simulink model "RL_TTS3_Controller_Blank"  (R2019b)
settings: Solver=FixedStepAuto  StartTime=0.0  StopTime=1900  FixedStep=0.01  RelTol=1e-3
PostLoadFcn:
  | if any(exist('dsrtsu_mdlpostloadfcn', 'file') ~= 0), dsrtsu_mdlpostloadfcn('Execute', bdroot); end
libraries: simulink x1
settings Model: DSRTSU_INTERNAL_RTI_VER=550  DSRTSU_INTERNAL_RTI_TYPE=rti1104  RTICANMMDATA=struct('GeneralSetupData',struct('modelroot','E:\Will\RemoteLabs\TTS3\HostPC','generalsettings',struct('filesettings',struct('destfolder',struct('Name','RTICANMM_FILES','Check',1),'buildfolder',struct('Name','.','Check',1),'AbsDestfolder',struct('Name','E:\Will\RemoteLabs\TTS3\HostPC\RTICANMM_FILES'),'AbsBuildfolder',struct('Name','E:\Will\RemoteLabs\TTS3\HostPC'))),'options',struct('addpaths',1,'rmpaths',1,'addtrcexclusion',true,'cannavigator',struct('checkmonitoring',0),'show_usrtrc',0,'use_usrtrc',0),'advanced',struct('options',ones(1,100)),'MPSetup',{{}},'RTI',struct('Type','RTI1104','Ver','7.13','Date','02-Nov-2019'),'modelname','TTS3_Controller_Test_OL','block','TTS3_Controller_Test_OL'))  DSRTSU_INTERNAL_RTIFPGA=150  Creator=whendrix  LastModifiedBy=Bart
settings OptimizationCC: BlockReduction=off  OptimizeBlockIOStorage=off  BufferReuse=off  GlobalBufferReuse=off  ExpressionFolding=off  LocalBlockOutputs=off  OptimizeDataStoreBuffers=off  BusAssignmentInplaceUpdate=off
settings DebuggingCC: BusObjectLabelMismatch=none
settings HardwareCC: ProdBitPerPointer=32  ProdBitPerSizeT=32  ProdBitPerPtrDiffT=32  ProdLargestAtomicInteger=Integer  ProdEndianess=BigEndian  ProdWordSize=32  ProdHWDeviceType=Custom Processor->Custom  TargetIntDivRoundTo=Zero  TargetEndianess=BigEndian  TargetHWDeviceType=Custom Processor->Custom
settings ModelReferenceCC: ModelReferenceNumInstancesAllowed=Single  ModelReferenceMinAlgLoopOccurrences=on
settings SFSimCC: MATLABDynamicMemAlloc=off  CustomCodeUndefinedFunction=UseInterfaceOnly
settings RTWCC: Description=dSPACE DS1104 Hardware Platform  SystemTargetFile=rti1104.tlc  MakeCommand=make_rti  TemplateMakefile=rti1104.tmf
settings CodeAppCC: MaxIdLength=63
settings STFCustomTargetCC: ParMdlRefBuildCompliant=on  SystemTargetFile=rti1104.tlc
settings GRTTargetCC: TargetLangStandard=C89/C90 (ANSI)  CompOptLevelCompliant=off  ConcurrentExecutionCompliant=off  CombineOutputUpdateFcns=off  MatFileLogging=off  CPPClassGenCompliant=off  UseToolchainInfoCompliant=off

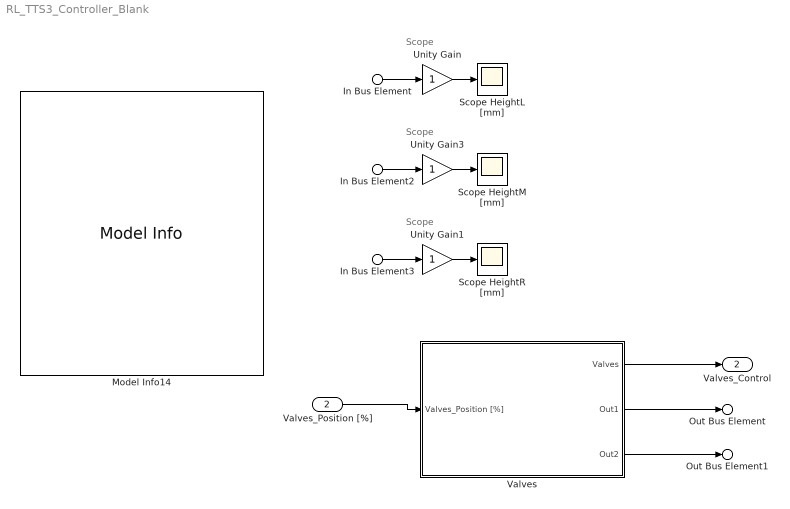
== system RL_TTS3_Controller_Blank ==
  note: Scope
  note: Scope
  note: Scope
  In Bus Element : Inport  PortName=Heights [mm]  Element=Left
  In Bus Element2 : Inport  PortName=Heights [mm]  Element=Middle
  In Bus Element3 : Inport  PortName=Heights [mm]  Element=Right
  Valves_Position [%] : Inport  Port=2  OutDataTypeStr=Bus: ValvesSOCI
  Model Info14 : simulink/Model-Wide Utilities/Model Info  Frame=on  DisplayStringWithTags=|  HorizontalTextAlignment=Left  LeftAlignmentValue=0.02
      | Start model for the "Three Tank"
      | experiment on the "Three Tank" setup.
      | Version: 1.0
      | 
      | 
      | INFORMATION
      | ----------------------
      | 
      | Unity Gain block before Scope is needed for
      | RemoteLabs compatebility. 
      | Do not modify or remove!
      | 
      | Pump range:
      | 0 to 0.102 [l/s]
      | 
      | The 5 Valves are labeled according 
      | to their position:
      | 
      |    LM  MR
      |      X     X
      |  X      X      X
      | LD    MD   RD
      | 
      | L = Left
      | M = Middle
      | R = Right
      | D = Down
  Scope HeightL [mm] : Scope
  Scope HeightM [mm] : Scope
  Scope HeightR [mm] : Scope
  Unity Gain : Gain
  Unity Gain1 : Gain
  Unity Gain3 : Gain
  Valves : Subsystem  TreatAsAtomicUnit=on
  Out Bus Element : Outport  VectorParamsAs1DForOutWhenUnconnected=off  PortName=Pumps [l/s]  Element=Left
  Out Bus Element1 : Outport  VectorParamsAs1DForOutWhenUnconnected=off  PortName=Pumps [l/s]  Element=Right
  Valves_Control : Outport  Port=2  OutDataTypeStr=Bus: ValvesSICO  VectorParamsAs1DForOutWhenUnconnected=off
  wires:
  Unity Gain3/1 -> Scope HeightM [mm]/1
  Unity Gain1/1 -> Scope HeightR [mm]/1
  In Bus Element/1 -> Unity Gain/1
  In Bus Element2/1 -> Unity Gain3/1
  In Bus Element3/1 -> Unity Gain1/1
  Valves/1(Valves) -> Valves_Control/1
  Valves_Position [%]/1 -> Valves/1(Valves_Position [%])
  Unity Gain/1 -> Scope HeightL [mm]/1
  Valves/2(Out1) -> Out Bus Element/1
  Valves/3(Out2) -> Out Bus Element1/1

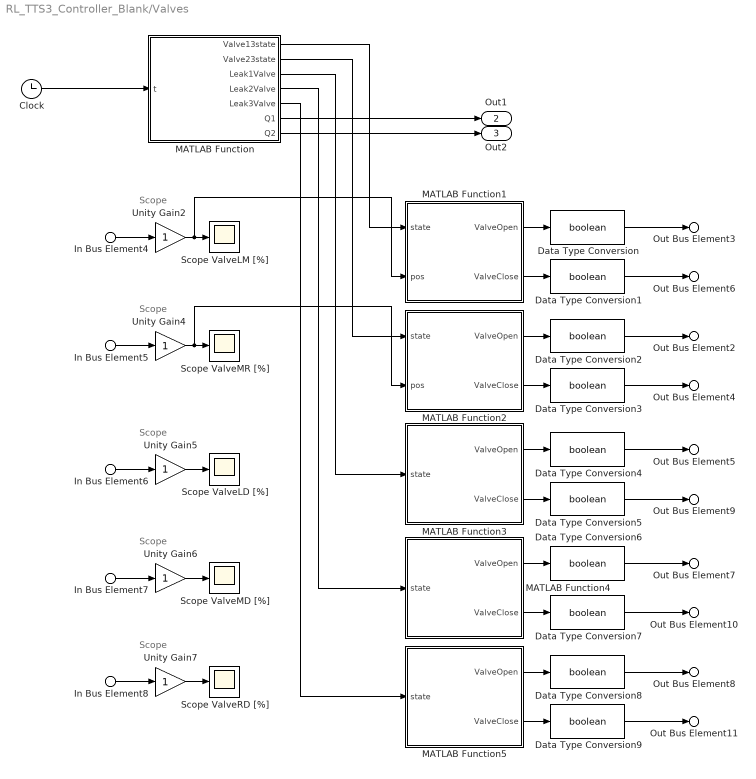
== system RL_TTS3_Controller_Blank/Valves ==
  note: Scope
  note: Scope
  note: Scope
  note: Scope
  note: Scope
  In Bus Element4 : Inport  PortName=Valves_Position [%]  Element=LeftMiddle
  In Bus Element5 : Inport  PortName=Valves_Position [%]  Element=MiddleRight
  In Bus Element6 : Inport  PortName=Valves_Position [%]  Element=LeftDown
  In Bus Element7 : Inport  PortName=Valves_Position [%]  Element=MiddleDown
  In Bus Element8 : Inport  PortName=Valves_Position [%]  Element=RightDown
  Clock : Clock
      settings: Decimation=100
  Data Type Conversion{,1..9} (10 alike) : DataTypeConversion  OutDataTypeStr=boolean
  MATLAB Function : MATLAB Function  TreatAsAtomicUnit=on
  MATLAB Function1 : MATLAB Function  TreatAsAtomicUnit=on
  MATLAB Function2 : MATLAB Function  TreatAsAtomicUnit=on
  MATLAB Function3 : MATLAB Function  TreatAsAtomicUnit=on
  MATLAB Function4 : MATLAB Function  TreatAsAtomicUnit=on
  MATLAB Function5 : MATLAB Function  TreatAsAtomicUnit=on
  Scope ValveLD [%] : Scope
  Scope ValveLM [%] : Scope
  Scope ValveMD [%] : Scope
  Scope ValveMR [%] : Scope
  Scope ValveRD [%] : Scope
  Unity Gain{2,4..7} (5 alike) : Gain
  Out Bus Element8 : Outport  VectorParamsAs1DForOutWhenUnconnected=off  PortName=Valves  Element=RightDown.Open
  Out Bus Element11 : Outport  VectorParamsAs1DForOutWhenUnconnected=off  PortName=Valves  Element=RightDown.Close
  Out Bus Element5 : Outport  VectorParamsAs1DForOutWhenUnconnected=off  PortName=Valves  Element=LeftDown.Open
  Out Bus Element9 : Outport  VectorParamsAs1DForOutWhenUnconnected=off  PortName=Valves  Element=LeftDown.Close
  Out Bus Element7 : Outport  VectorParamsAs1DForOutWhenUnconnected=off  PortName=Valves  Element=MiddleDown.Open
  Out Bus Element10 : Outport  VectorParamsAs1DForOutWhenUnconnected=off  PortName=Valves  Element=MiddleDown.Close
  Out Bus Element2 : Outport  VectorParamsAs1DForOutWhenUnconnected=off  PortName=Valves  Element=MiddleRight.Open
  Out Bus Element4 : Outport  VectorParamsAs1DForOutWhenUnconnected=off  PortName=Valves  Element=MiddleRight.Close
  Out Bus Element3 : Outport  VectorParamsAs1DForOutWhenUnconnected=off  PortName=Valves  Element=LeftMiddle.Open
  Out Bus Element6 : Outport  VectorParamsAs1DForOutWhenUnconnected=off  PortName=Valves  Element=LeftMiddle.Close
  Out1 : Outport  Port=2
  Out2 : Outport  Port=3
  wires:
  In Bus Element5/1 -> Unity Gain4/1
  In Bus Element4/1 -> Unity Gain2/1
  In Bus Element7/1 -> Unity Gain6/1
  Unity Gain6/1 -> Scope ValveMD [%]/1
  In Bus Element6/1 -> Unity Gain5/1
  In Bus Element8/1 -> Unity Gain7/1
  Unity Gain7/1 -> Scope ValveRD [%]/1
  Unity Gain4/1 -> MATLAB Function2/2(pos), Scope ValveMR [%]/1
  Unity Gain5/1 -> Scope ValveLD [%]/1
  Unity Gain2/1 -> MATLAB Function1/2(pos), Scope ValveLM [%]/1
  Data Type Conversion/1 -> Out Bus Element3/1
  Data Type Conversion1/1 -> Out Bus Element6/1
  Data Type Conversion2/1 -> Out Bus Element2/1
  Data Type Conversion3/1 -> Out Bus Element4/1
  Data Type Conversion4/1 -> Out Bus Element5/1
  Data Type Conversion5/1 -> Out Bus Element9/1
  Data Type Conversion6/1 -> Out Bus Element7/1
  Data Type Conversion7/1 -> Out Bus Element10/1
  Data Type Conversion8/1 -> Out Bus Element8/1
  Data Type Conversion9/1 -> Out Bus Element11/1
  Clock/1 -> MATLAB Function/1(t)
  MATLAB Function1/1(ValveOpen) -> Data Type Conversion/1
  MATLAB Function1/2(ValveClose) -> Data Type Conversion1/1
  MATLAB Function/1(Valve13state) -> MATLAB Function1/1(state)
  MATLAB Function2/1(ValveOpen) -> Data Type Conversion2/1
  MATLAB Function2/2(ValveClose) -> Data Type Conversion3/1
  MATLAB Function/2(Valve23state) -> MATLAB Function2/1(state)
  MATLAB Function3/1(ValveOpen) -> Data Type Conversion4/1
  MATLAB Function3/2(ValveClose) -> Data Type Conversion5/1
  MATLAB Function/3(Leak1Valve) -> MATLAB Function3/1(state)
  MATLAB Function4/1(ValveOpen) -> Data Type Conversion6/1
  MATLAB Function4/2(ValveClose) -> Data Type Conversion7/1
  MATLAB Function5/1(ValveOpen) -> Data Type Conversion8/1
  MATLAB Function5/2(ValveClose) -> Data Type Conversion9/1
  MATLAB Function/5(Leak3Valve) -> MATLAB Function5/1(state)
  MATLAB Function/4(Leak2Valve) -> MATLAB Function4/1(state)
  MATLAB Function/6(Q1) -> Out1/1
  MATLAB Function/7(Q2) -> Out2/1

== matlab function RL_TTS3_Controller_Blank/Valves/MATLAB Function1 ==
  data: state input; ValveOpen output; ValveClose output; pos input
function [ValveOpen, ValveClose] = Valve13(state,pos)
statepos = state(2);
state = state(1);

switch state
    case 0
        ValveOpen = false;
        ValveClose = true;
    case 1
        if(pos<statepos)
            ValveOpen = true;
            ValveClose = false;
        elseif(pos>=statepos)
            % semiopen poistion
            ValveOpen = false;
            ValveClose = false;
        end
    case 2
        ValveOpen = false;
        ValveClose = false;
    case 3
        ValveOpen = true;
        ValveClose = false;
    otherwise
        0;
end
end

== matlab function RL_TTS3_Controller_Blank/Valves/MATLAB Function ==
  data: t input; Valve13state output; Valve23state output; Leak1Valve output; Leak2Valve output; Leak3Valve output; Q1 output; Q2 output
function [Valve13state,Valve23state, Leak1Valve, Leak2Valve, Leak3Valve, Q1,Q2] = FSM(t)

percentageOpen = 20;
tankToTest = 2;

% state nr:
% 0: all valves closed
% 1: let valves go from a initial position to a percentage
% 2: do nothing
% 3: all valves 100% open

if(tankToTest==1)
    if(t<=90)
        % state 0
        Valve13state = [0 0];
        Valve23state = [0 0];
        Leak1Valve = 0;
        Leak2Valve = 0;
        Leak3Valve = 0;
        Q1 = 0.1;
        Q2 = 0;
        
    elseif (t>90 && t<=100)
        % state 1
        Valve13state = [1 percentageOpen];
        Valve23state = [1 0];
        Leak1Valve = 1;
        Leak2Valve = 1;
        Leak3Valve = 1;
        Q1 = 0;
        Q2 = 0;
        
    elseif (t>100)
        % state 2: observe
        Valve13state = [2 0];
        Valve23state = [2 0];
        Leak1Valve = 2;
        Leak2Valve = 2;
        Leak3Valve = 2;
        Q1 = 0;
        Q2 = 0;
    end
    
    
end

if(tankToTest==2)
    if(t<=80)
        % state 0
        Valve13state = [0 0];
        Valve23state = [0 0];
        Leak1Valve = 0;
        Leak2Valve = 0;
        Leak3Valve = 0;
        Q1 = 0;
        Q2 = 0.1;
        
    elseif (t>80 && t<=90)
        % state 1
        Valve13state = [1 0];
        Valve23state = [1 percentageOpen];
        Leak1Valve = 1;
        Leak2Valve = 1;
        Leak3Valve = 1;
        Q1 = 0;
        Q2 = 0;
        
    elseif (t>90)
        % state 2: observe
        Valve13state = [2 0];
        Valve23state = [2 0];
        Leak1Valve = 2;
        Leak2Valve = 2;
        Leak3Valve = 2;
        Q1 = 0;
        Q2 = 0;
    end
    
    
end
end

== matlab function RL_TTS3_Controller_Blank/Valves/MATLAB Function2 ==
  data: state input; ValveOpen output; ValveClose output; pos input
function [ValveOpen, ValveClose] = Valve32(state,pos)
statepos = state(2);
state = state(1);

switch state
    case 0
        ValveOpen = false;
        ValveClose = true;
    case 1
        if(pos<statepos)
            ValveOpen = true;
            ValveClose = false;
        elseif(pos>=statepos)
            % semiopen poistion
            ValveOpen = false;
            ValveClose = false;
        end
    case 2
        ValveOpen = false;
        ValveClose = false;
    case 3
        ValveOpen = true;
        ValveClose = false;
    otherwise
        0;
end
end

== matlab function RL_TTS3_Controller_Blank/Valves/MATLAB Function3 ==
  data: state input; ValveOpen output; ValveClose output
function [ValveOpen, ValveClose] = Leak1Valve(state)
switch state
    case 0
        ValveOpen = false;
        ValveClose = true;
    case 1
        ValveOpen = false;
        ValveClose = true;
    case 2
        ValveOpen = false;
        ValveClose = true;
    case 3
        ValveOpen = true;
        ValveClose = false;
    otherwise
        0;
end
end

== matlab function RL_TTS3_Controller_Blank/Valves/MATLAB Function4 ==
  data: state input; ValveOpen output; ValveClose output
function [ValveOpen, ValveClose] = Leak2Valve(state)
switch state
    case 0
        ValveOpen = false;
        ValveClose = true;
    case 1
        ValveOpen = false;
        ValveClose = true;
    case 2
        ValveOpen = false;
        ValveClose = true;
    case 3
        ValveOpen = true;
        ValveClose = false;
    otherwise
        0;
end
end

== matlab function RL_TTS3_Controller_Blank/Valves/MATLAB Function5 ==
  data: state input; ValveOpen output; ValveClose output
function [ValveOpen, ValveClose] = Leak3Valve(state)
switch state
    case 0
        ValveOpen = false;
        ValveClose = true;
    case 1
        ValveOpen = false;
        ValveClose = true;
    case 2
        ValveOpen = false;
        ValveClose = true;
    case 3
        ValveOpen = true;
        ValveClose = false;
    otherwise
        0;
end
end
